simulink library "VLS_Standard_Library"  (R2020b)
settings: Solver=VariableStepAuto  StartTime=0.0  StopTime=10.0  RelTol=1e-3
libraries: simulink x11
Description:
  | VLS Standard Library
  | Version: 1.1.0
settings Model: Creator=mchawa  LastModifiedBy=mchawa
settings DataIOCC: ReturnWorkspaceOutputs=off
settings DebuggingCC: ArithmeticOperatorsInVariantConditions=warning
settings SFSimCC: SimUseLocalCustomCode=off  CustomCodeUndefinedFunction=UseInterfaceOnly
settings RTWCC: RTWUseLocalCustomCode=off

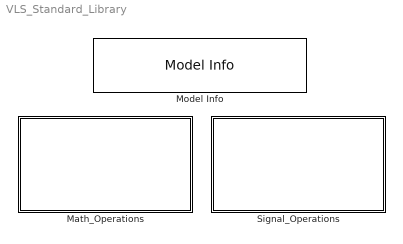
== system VLS_Standard_Library ==
  Math_Operations : Subsystem
  Model Info : simulink/Model-Wide Utilities/Model Info  Frame=on  DisplayStringWithTags=|  HorizontalTextAlignment=Center  LeftAlignmentValue=0.5
      | Model Info
      | Name: %<ModelName>
      | Description: %<Description>
  Signal_Operations : Subsystem

== system VLS_Standard_Library/Math_Operations ==
  SimpleSecureDivision : Subsystem

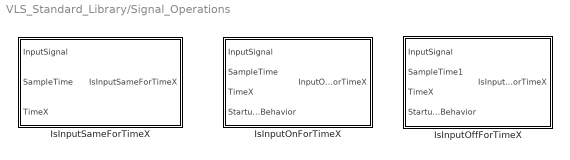
== system VLS_Standard_Library/Signal_Operations ==
  IsInputOffForTimeX : Subsystem
  IsInputOnForTimeX : Subsystem
  IsInputSameForTimeX : Subsystem

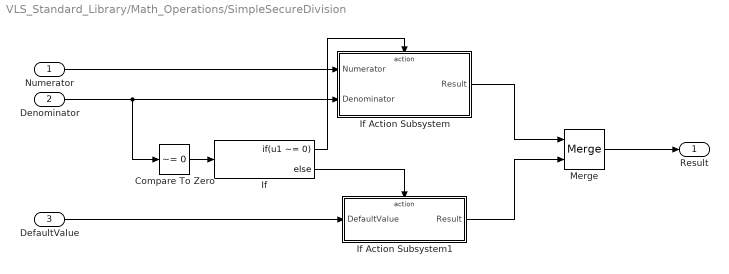
== system VLS_Standard_Library/Math_Operations/SimpleSecureDivision ==
  Numerator : Inport
  Denominator : Inport  Port=2
  DefaultValue : Inport  Port=3
  Compare To Zero : simulink/Logic and Bit Operations/Compare To Zero  relop=~=  OutDataTypeStr=boolean
  If : If  IfExpression=u1 ~= 0
  If Action Subsystem : Subsystem  TreatAsAtomicUnit=on
  If Action Subsystem1 : Subsystem  TreatAsAtomicUnit=on
  Merge : Merge
  Result : Outport  VectorParamsAs1DForOutWhenUnconnected=off
  wires:
  Numerator/1 -> If Action Subsystem/1(Numerator)
  If/2 -> If Action Subsystem1/Action
  Denominator/1 -> If Action Subsystem/2(Denominator), Compare To Zero/1
  If Action Subsystem/1(Result) -> Merge/1
  If Action Subsystem1/1(Result) -> Merge/2
  Merge/1 -> Result/1
  DefaultValue/1 -> If Action Subsystem1/1(DefaultValue)
  If/1 -> If Action Subsystem/Action
  Compare To Zero/1 -> If/1

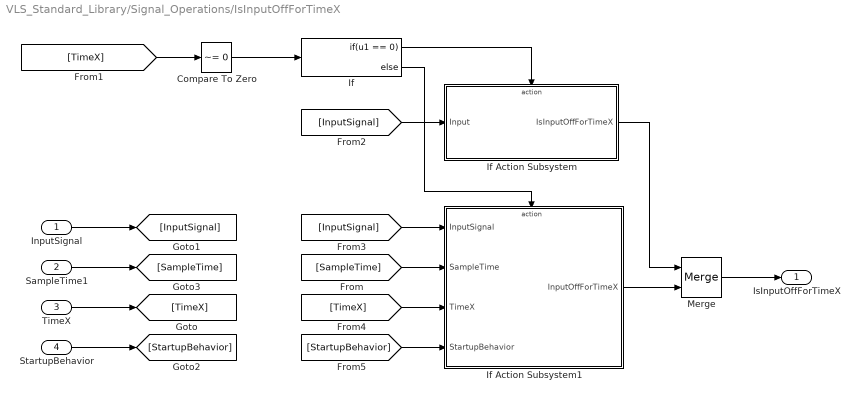
== system VLS_Standard_Library/Signal_Operations/IsInputOffForTimeX ==
  InputSignal : Inport
  SampleTime1 : Inport  Port=2
  TimeX : Inport  Port=3
  StartupBehavior : Inport  Port=4
  Compare To Zero : simulink/Logic and Bit Operations/Compare To Zero  relop=~=  OutDataTypeStr=boolean
  If : If  IfExpression=u1 == 0
  If Action Subsystem : Subsystem  TreatAsAtomicUnit=on
  If Action Subsystem1 : Subsystem  TreatAsAtomicUnit=on
  Merge : Merge
  IsInputOffForTimeX : Outport  VectorParamsAs1DForOutWhenUnconnected=off
  wires:
  Compare To Zero/1 -> If/1
  Merge/1 -> IsInputOffForTimeX/1
  If Action Subsystem1/1(InputOffForTimeX) -> Merge/2
  If Action Subsystem/1(IsInputOffForTimeX) -> Merge/1
  [TimeX] -> If Action Subsystem1/3(TimeX)
  [TimeX] -> Compare To Zero/1
  If/2 -> If Action Subsystem1/Action
  [InputSignal] -> If Action Subsystem1/1(InputSignal)
  [InputSignal] -> If Action Subsystem/1(Input)
  If/1 -> If Action Subsystem/Action
  StartupBehavior/1 -> [StartupBehavior]
  TimeX/1 -> [TimeX]
  InputSignal/1 -> [InputSignal]
  SampleTime1/1 -> [SampleTime]
  [SampleTime] -> If Action Subsystem1/2(SampleTime)
  [StartupBehavior] -> If Action Subsystem1/4(StartupBehavior)

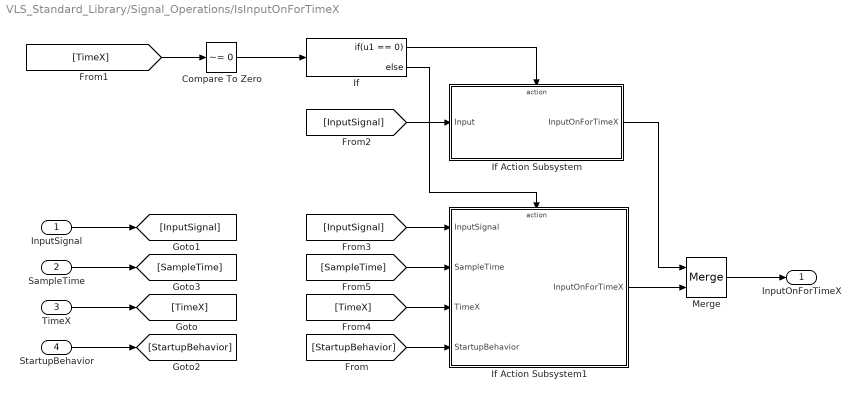
== system VLS_Standard_Library/Signal_Operations/IsInputOnForTimeX ==
  InputSignal : Inport
  SampleTime : Inport  Port=2
  TimeX : Inport  Port=3
  StartupBehavior : Inport  Port=4
  Compare To Zero : simulink/Logic and Bit Operations/Compare To Zero  relop=~=  OutDataTypeStr=boolean
  If : If  IfExpression=u1 == 0
  If Action Subsystem : Subsystem  TreatAsAtomicUnit=on
  If Action Subsystem1 : Subsystem  TreatAsAtomicUnit=on
  Merge : Merge
  InputOnForTimeX : Outport  VectorParamsAs1DForOutWhenUnconnected=off
  wires:
  If/1 -> If Action Subsystem/Action
  InputSignal/1 -> [InputSignal]
  [InputSignal] -> If Action Subsystem/1(Input)
  [InputSignal] -> If Action Subsystem1/1(InputSignal)
  If/2 -> If Action Subsystem1/Action
  TimeX/1 -> [TimeX]
  [TimeX] -> Compare To Zero/1
  [TimeX] -> If Action Subsystem1/3(TimeX)
  If Action Subsystem/1(InputOnForTimeX) -> Merge/1
  If Action Subsystem1/1(InputOnForTimeX) -> Merge/2
  Merge/1 -> InputOnForTimeX/1
  Compare To Zero/1 -> If/1
  StartupBehavior/1 -> [StartupBehavior]
  [StartupBehavior] -> If Action Subsystem1/4(StartupBehavior)
  SampleTime/1 -> [SampleTime]
  [SampleTime] -> If Action Subsystem1/2(SampleTime)

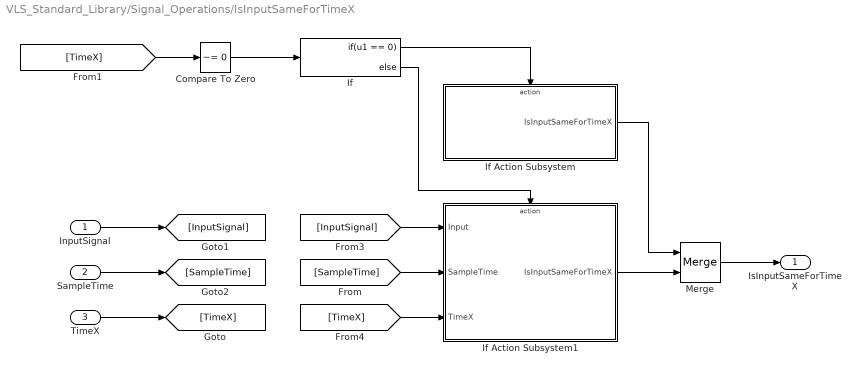
== system VLS_Standard_Library/Signal_Operations/IsInputSameForTimeX ==
  InputSignal : Inport
  SampleTime : Inport  Port=2
  TimeX : Inport  Port=3
  Compare To Zero : simulink/Logic and Bit Operations/Compare To Zero  relop=~=  OutDataTypeStr=boolean
  If : If  IfExpression=u1 == 0
  If Action Subsystem : Subsystem  TreatAsAtomicUnit=on
  If Action Subsystem1 : Subsystem  TreatAsAtomicUnit=on
  Merge : Merge
  IsInputSameForTimeX : Outport  VectorParamsAs1DForOutWhenUnconnected=off
  wires:
  Compare To Zero/1 -> If/1
  Merge/1 -> IsInputSameForTimeX/1
  If Action Subsystem1/1(IsInputSameForTimeX) -> Merge/2
  If Action Subsystem/1(IsInputSameForTimeX) -> Merge/1
  [TimeX] -> If Action Subsystem1/3(TimeX)
  [TimeX] -> Compare To Zero/1
  TimeX/1 -> [TimeX]
  If/2 -> If Action Subsystem1/Action
  [InputSignal] -> If Action Subsystem1/1(Input)
  InputSignal/1 -> [InputSignal]
  If/1 -> If Action Subsystem/Action
  SampleTime/1 -> [SampleTime]
  [SampleTime] -> If Action Subsystem1/2(SampleTime)

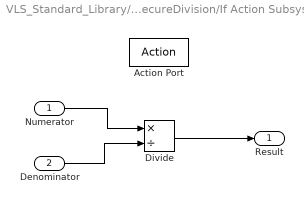
== system VLS_Standard_Library/Math_Operations/SimpleSecureDivision/If Action Subsystem ==
  Numerator : Inport
  Denominator : Inport  Port=2
  Action Port : ActionPort
  Divide : Product  Inputs=*/  OutDataTypeStr=Inherit: Inherit via back propagation
  Result : Outport  VectorParamsAs1DForOutWhenUnconnected=off
  wires:
  Divide/1 -> Result/1
  Numerator/1 -> Divide/1
  Denominator/1 -> Divide/2

== system VLS_Standard_Library/Math_Operations/SimpleSecureDivision/If Action Subsystem1 ==
  DefaultValue : Inport
  Action Port : ActionPort
  Result : Outport  VectorParamsAs1DForOutWhenUnconnected=off
  wires:
  DefaultValue/1 -> Result/1

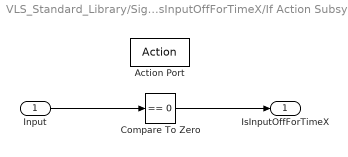
== system VLS_Standard_Library/Signal_Operations/IsInputOffForTimeX/If Action Subsystem ==
  Input : Inport
  Action Port : ActionPort
  Compare To Zero : simulink/Logic and Bit Operations/Compare To Zero  relop===  OutDataTypeStr=boolean
  IsInputOffForTimeX : Outport  VectorParamsAs1DForOutWhenUnconnected=off
  wires:
  Compare To Zero/1 -> IsInputOffForTimeX/1
  Input/1 -> Compare To Zero/1

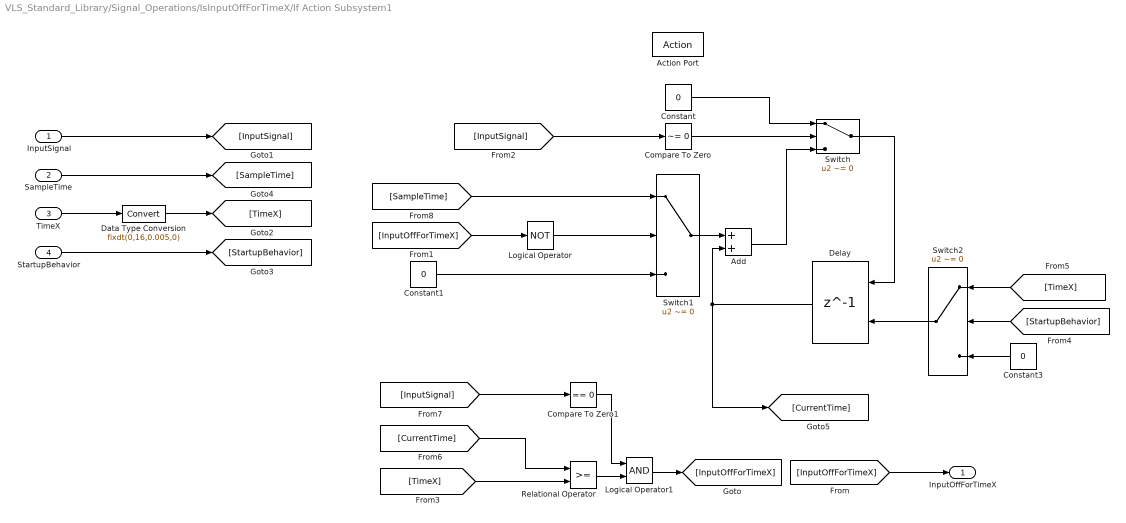
== system VLS_Standard_Library/Signal_Operations/IsInputOffForTimeX/If Action Subsystem1 ==
  InputSignal : Inport
  SampleTime : Inport  Port=2
  TimeX : Inport  Port=3
  StartupBehavior : Inport  Port=4
  Action Port : ActionPort  ActionPortLabel=else
  Add : Sum
  Compare To Zero : simulink/Logic and Bit Operations/Compare To Zero  relop=~=  OutDataTypeStr=boolean
  Compare To Zero1 : simulink/Logic and Bit Operations/Compare To Zero  relop===  OutDataTypeStr=boolean
  Constant : Constant  Value=0  OutDataTypeStr=Inherit: Inherit via back propagation
  Constant1 : Constant  Value=0  OutDataTypeStr=Inherit: Inherit via back propagation
  Constant3 : Constant  Value=0  OutDataTypeStr=Inherit: Inherit via back propagation
  Data Type Conversion : DataTypeConversion  OutDataTypeStr=fixdt(0,16,0.005,0)  SaturateOnIntegerOverflow=on
  Delay : Delay  DelayLength=1  InitialConditionSource=Input port
      settings: InputPortMap=u0,p4
  Logical Operator : Logic  Operator=NOT  AllPortsSameDT=off  OutDataTypeStr=boolean
  Logical Operator1 : Logic  AllPortsSameDT=off  OutDataTypeStr=boolean
  Relational Operator : RelationalOperator  OutDataTypeStr=boolean  RndMeth=Simplest
  Switch : Switch  Criteria=u2 ~= 0
  Switch1 : Switch  Criteria=u2 ~= 0
  Switch2 : Switch  Criteria=u2 ~= 0
  InputOffForTimeX : Outport  VectorParamsAs1DForOutWhenUnconnected=off
  wires:
  [TimeX] -> Switch2/1
  Switch2/1 -> Delay/2
  [StartupBehavior] -> Switch2/2
  [SampleTime] -> Switch1/1
  SampleTime/1 -> [SampleTime]
  Constant3/1 -> Switch2/3
  Constant/1 -> Switch/1
  TimeX/1 -> Data Type Conversion/1
  Relational Operator/1 -> Logical Operator1/2
  Delay/1 -> [CurrentTime], Add/2
  Switch/1 -> Delay/1
  Data Type Conversion/1 -> [TimeX]
  StartupBehavior/1 -> [StartupBehavior]
  [CurrentTime] -> Relational Operator/1
  [TimeX] -> Relational Operator/2
  Compare To Zero/1 -> Switch/2
  [InputOffForTimeX] -> Logical Operator/1
  Add/1 -> Switch/3
  Switch1/1 -> Add/1
  Logical Operator/1 -> Switch1/2
  InputSignal/1 -> [InputSignal]
  Constant1/1 -> Switch1/3
  [InputSignal] -> Compare To Zero/1
  Logical Operator1/1 -> [InputOffForTimeX]
  [InputOffForTimeX] -> InputOffForTimeX/1
  [InputSignal] -> Compare To Zero1/1
  Compare To Zero1/1 -> Logical Operator1/1

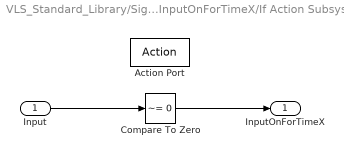
== system VLS_Standard_Library/Signal_Operations/IsInputOnForTimeX/If Action Subsystem ==
  Input : Inport
  Action Port : ActionPort  ActionPortLabel=if { }
  Compare To Zero : simulink/Logic and Bit Operations/Compare To Zero  relop=~=  OutDataTypeStr=boolean
  InputOnForTimeX : Outport  VectorParamsAs1DForOutWhenUnconnected=off
  wires:
  Input/1 -> Compare To Zero/1
  Compare To Zero/1 -> InputOnForTimeX/1

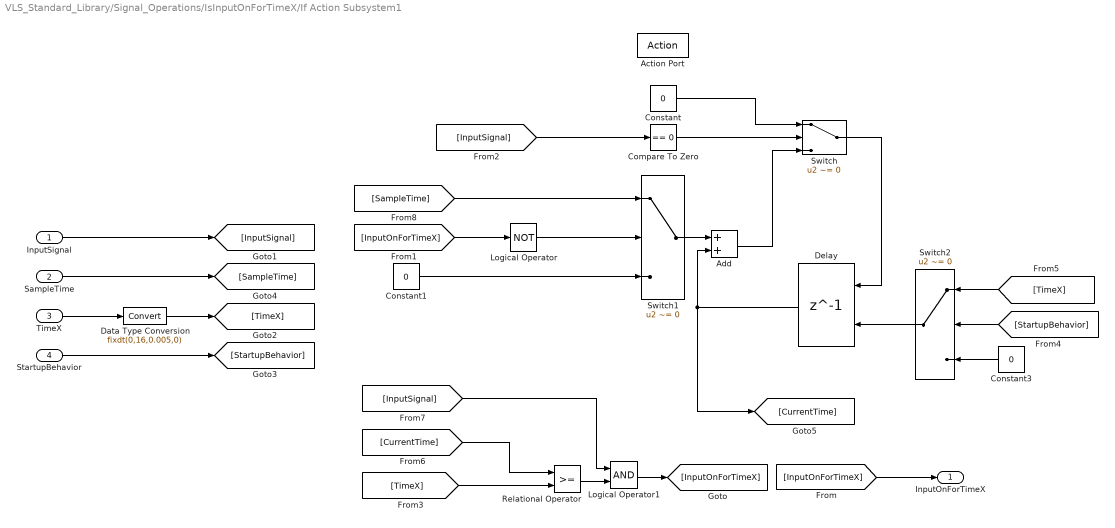
== system VLS_Standard_Library/Signal_Operations/IsInputOnForTimeX/If Action Subsystem1 ==
  InputSignal : Inport
  SampleTime : Inport  Port=2
  TimeX : Inport  Port=3
  StartupBehavior : Inport  Port=4
  Action Port : ActionPort  ActionPortLabel=else { }
  Add : Sum
  Compare To Zero : simulink/Logic and Bit Operations/Compare To Zero  relop===  OutDataTypeStr=boolean
  Constant : Constant  Value=0  OutDataTypeStr=Inherit: Inherit via back propagation
  Constant1 : Constant  Value=0  OutDataTypeStr=Inherit: Inherit via back propagation
  Constant3 : Constant  Value=0  OutDataTypeStr=Inherit: Inherit via back propagation
  Data Type Conversion : DataTypeConversion  OutDataTypeStr=fixdt(0,16,0.005,0)  SaturateOnIntegerOverflow=on
  Delay : Delay  DelayLength=1  InitialConditionSource=Input port
      settings: InputPortMap=u0,p4
  Logical Operator : Logic  Operator=NOT  AllPortsSameDT=off  OutDataTypeStr=boolean
  Logical Operator1 : Logic  AllPortsSameDT=off  OutDataTypeStr=boolean
  Relational Operator : RelationalOperator  OutDataTypeStr=boolean  RndMeth=Simplest
  Switch : Switch  Criteria=u2 ~= 0
  Switch1 : Switch  Criteria=u2 ~= 0
  Switch2 : Switch  Criteria=u2 ~= 0
  InputOnForTimeX : Outport  VectorParamsAs1DForOutWhenUnconnected=off
  wires:
  [InputOnForTimeX] -> Logical Operator/1
  [InputOnForTimeX] -> InputOnForTimeX/1
  Constant1/1 -> Switch1/3
  Switch1/1 -> Add/1
  Add/1 -> Switch/3
  Compare To Zero/1 -> Switch/2
  Constant/1 -> Switch/1
  Delay/1 -> [CurrentTime], Add/2
  TimeX/1 -> Data Type Conversion/1
  Switch/1 -> Delay/1
  Logical Operator/1 -> Switch1/2
  Relational Operator/1 -> Logical Operator1/2
  Logical Operator1/1 -> [InputOnForTimeX]
  Switch2/1 -> Delay/2
  [StartupBehavior] -> Switch2/2
  InputSignal/1 -> [InputSignal]
  [InputSignal] -> Compare To Zero/1
  Data Type Conversion/1 -> [TimeX]
  [TimeX] -> Relational Operator/2
  StartupBehavior/1 -> [StartupBehavior]
  SampleTime/1 -> [SampleTime]
  [CurrentTime] -> Relational Operator/1
  [InputSignal] -> Logical Operator1/1
  [SampleTime] -> Switch1/1
  [TimeX] -> Switch2/1
  Constant3/1 -> Switch2/3

== system VLS_Standard_Library/Signal_Operations/IsInputSameForTimeX/If Action Subsystem ==
  Action Port : ActionPort
  Constant : Constant  Value=true  OutDataTypeStr=boolean
  IsInputSameForTimeX : Outport  VectorParamsAs1DForOutWhenUnconnected=off
  wires:
  Constant/1 -> IsInputSameForTimeX/1

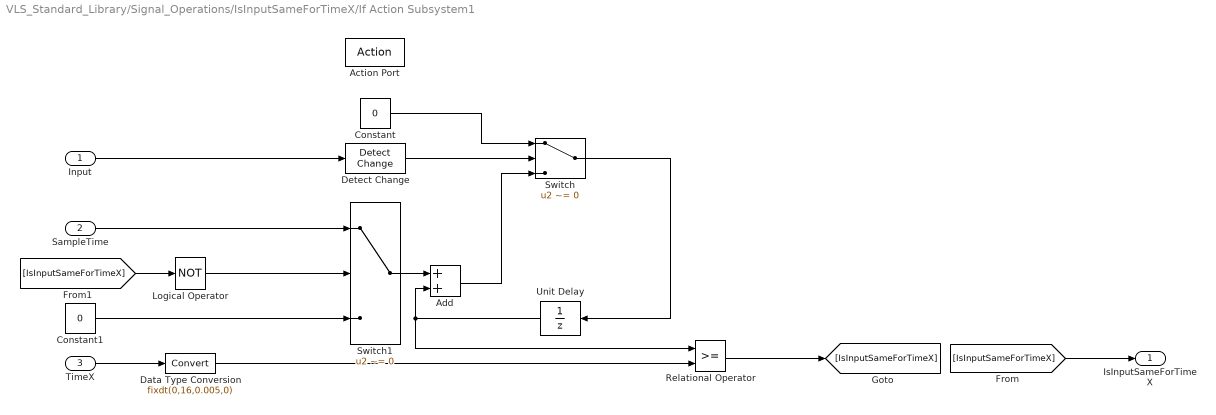
== system VLS_Standard_Library/Signal_Operations/IsInputSameForTimeX/If Action Subsystem1 ==
  Input : Inport
  SampleTime : Inport  Port=2
  TimeX : Inport  Port=3
  Action Port : ActionPort
  Add : Sum
  Constant : Constant  Value=0  OutDataTypeStr=Inherit: Inherit via back propagation
  Constant1 : Constant  Value=0  OutDataTypeStr=Inherit: Inherit via back propagation
  Data Type Conversion : DataTypeConversion  OutDataTypeStr=fixdt(0,16,0.005,0)  SaturateOnIntegerOverflow=on
  Detect Change : simulink/Logic and Bit Operations/Detect Change  vinit=0  OutDataTypeStr=boolean
  Logical Operator : Logic  Operator=NOT  AllPortsSameDT=off  OutDataTypeStr=boolean
  Relational Operator : RelationalOperator  OutDataTypeStr=boolean  RndMeth=Simplest
  Switch : Switch  Criteria=u2 ~= 0
  Switch1 : Switch  Criteria=u2 ~= 0
  Unit Delay : UnitDelay  SampleTime=-1  HasFrameUpgradeWarning=on
  IsInputSameForTimeX : Outport  VectorParamsAs1DForOutWhenUnconnected=off
  wires:
  TimeX/1 -> Data Type Conversion/1
  Input/1 -> Detect Change/1
  Unit Delay/1 -> Add/2, Relational Operator/1
  Constant/1 -> Switch/1
  Detect Change/1 -> Switch/2
  Add/1 -> Switch/3
  Switch/1 -> Unit Delay/1
  Switch1/1 -> Add/1
  SampleTime/1 -> Switch1/1
  Logical Operator/1 -> Switch1/2
  Constant1/1 -> Switch1/3
  [IsInputSameForTimeX] -> IsInputSameForTimeX/1
  Data Type Conversion/1 -> Relational Operator/2
  [IsInputSameForTimeX] -> Logical Operator/1
  Relational Operator/1 -> [IsInputSameForTimeX]
